simulink model "Final_motores"  (R2020b)
settings: Solver=VariableStepAuto  StartTime=0.0  StopTime=10.0  MinStep=2e-6  RelTol=1e-3
model workspace (MAT data in the model file):
  potencia = 0.1
values from neighbouring files (symbols this model uses):
  b = 1.5e-5    (= 1.5e-05)    [Var_PF.m]
  Jl = Jl/100^2/1000    (= 0.00048022)    [Var_PF.m]
  Ke = Ke*60/(2*pi)    (= 131.78029288)    [Var_PF.m]
  Kt = Kt/100    (= 0.133)    [Var_PF.m]
  La = 1.4/1000    (= 0.0014)    [Var_PF.m]
  Ra = 0.4    [Var_PF.m]
undefined symbols (not defined in the file or in its folder): B, ba, C_f, DiscIntNeverNeededParam, f_mues, gama, Ksa, Ksia, Kto, Kwo, mult, ohmega_obser, ohmega_pos, r, R, R_f, time_MV, Vmax_controlador, Vmax_salida, w_ia
libraries: dspfdesign x3, commchan3 x3, mcbcontrolslib x2, simulink x1, dspstat3 x1
settings Model: Creator=GoniR  LastModifiedBy=GoniR

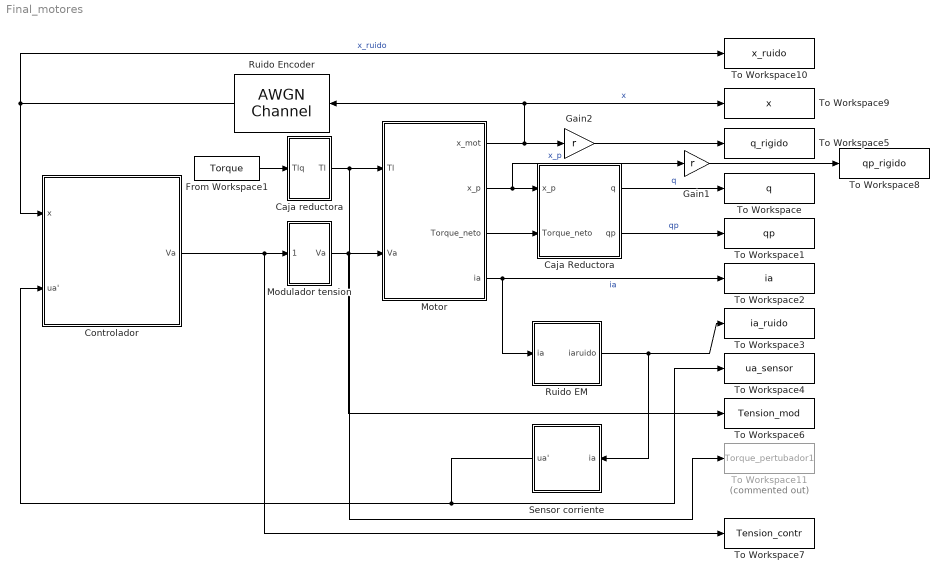
== system Final_motores ==
  Caja Reductora : Subsystem
  Caja reductora : Subsystem
  Controlador : Subsystem
  From Workspace1 : FromWorkspace  VariableName=Torque
  Gain1 : Gain  Gain=r
  Gain2 : Gain  Gain=r
  Modulador tension : Subsystem
  Motor : Subsystem
  Ruido EM : Subsystem
  Ruido Encoder : commchan3/AWGN Channel  InputProcessing=Columns as channels (frame based)  seed=67  noiseMode=Variance from mask  EbNodB=10  EsNodB=30  SNRdB=30  bitsPerSym=1  Ps=1  Tsym=1  variance=((1/(5000)*2*pi /360)/2)^2
  Sensor corriente : Subsystem
  To Workspace : ToWorkspace  VariableName=q  SaveFormat=Timeseries  SampleTime=-1
  To Workspace1 : ToWorkspace  VariableName=qp  SaveFormat=Timeseries  SampleTime=-1
  To Workspace10 : ToWorkspace  VariableName=x_ruido  SaveFormat=Timeseries  SampleTime=-1
  To Workspace11 : ToWorkspace  Commented=on  VariableName=Torque_pertubador1  SaveFormat=Timeseries  SampleTime=-1
  To Workspace2 : ToWorkspace  VariableName=ia  SaveFormat=Timeseries  SampleTime=-1
  To Workspace3 : ToWorkspace  VariableName=ia_ruido  SaveFormat=Timeseries  SampleTime=-1
  To Workspace4 : ToWorkspace  VariableName=ua_sensor  SaveFormat=Timeseries  SampleTime=-1
  To Workspace5 : ToWorkspace  VariableName=q_rigido  SaveFormat=Timeseries  SampleTime=-1
  To Workspace6 : ToWorkspace  VariableName=Tension_mod  SaveFormat=Timeseries  SampleTime=-1
  To Workspace7 : ToWorkspace  VariableName=Tension_contr  SaveFormat=Timeseries  SampleTime=-1
  To Workspace8 : ToWorkspace  VariableName=qp_rigido  SaveFormat=Timeseries  SampleTime=-1
  To Workspace9 : ToWorkspace  VariableName=x  SaveFormat=Timeseries  SampleTime=-1
  wires:
  Motor/4(ia) -> Ruido EM/1(ia), To Workspace2/1  "ia"
  Controlador/1(Va) -> To Workspace7/1, Modulador tension/1(Va*)
  Caja reductora/1(Tl) -> To Workspace11/1, Motor/1(Tl)
  Modulador tension/1(Va) -> To Workspace6/1, Motor/2(Va)
  Motor/2(x_p) -> Gain1/1, Caja Reductora/1(x_p)  "x_p"
  Sensor corriente/1(ua') -> Controlador/2(ua'), To Workspace4/1
  Caja Reductora/1(q) -> To Workspace/1  "q"
  Caja Reductora/2(qp) -> To Workspace1/1  "qp"
  Ruido EM/1(iaruido) -> Sensor corriente/1(ia), To Workspace3/1
  Motor/3(Torque_neto) -> Caja Reductora/2(Torque_neto)
  Motor/1(x_mot) -> Ruido Encoder/1, To Workspace9/1, Gain2/1  "x"
  Gain2/1 -> To Workspace5/1
  From Workspace1/1 -> Caja reductora/1(Tlq)
  Ruido Encoder/1 -> To Workspace10/1, Controlador/1(x)  "x_ruido"
  Gain1/1 -> To Workspace8/1

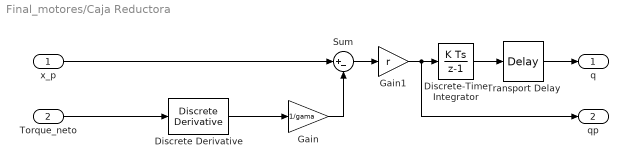
== system Final_motores/Caja Reductora ==
  x_p : Inport
  Torque_neto : Inport  Port=2
  Discrete Derivative : simulink/Discrete/Discrete Derivative  gainval=1.0  ICPrevScaledInput=0.0  OutMin=[]  OutMax=[]  OutDataType=fixdt(1, 16)  OutScaling=2^-10  DoSatur=off
  Discrete-Time Integrator : DiscreteIntegrator  SampleTime=-1  ICPrevOutput=DiscIntNeverNeededParam  ICPrevScaledInput=DiscIntNeverNeededParam
  Gain : Gain  Gain=1/gama
  Gain1 : Gain  Gain=r
  Sum : Sum  Inputs=|+-
  Transport Delay : TransportDelay  DelayTime=1e-6
  q : Outport
  qp : Outport  Port=2
  wires:
  Gain/1 -> Sum/2
  Torque_neto/1 -> Discrete Derivative/1
  Discrete Derivative/1 -> Gain/1
  x_p/1 -> Sum/1
  Sum/1 -> Gain1/1
  Discrete-Time Integrator/1 -> Transport Delay/1
  Transport Delay/1 -> q/1
  Gain1/1 -> qp/1, Discrete-Time Integrator/1

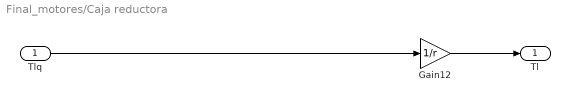
== system Final_motores/Caja reductora ==
  Tlq : Inport
  Gain12 : Gain  Gain=1/r
  Tl : Outport
  wires:
  Tlq/1 -> Gain12/1
  Gain12/1 -> Tl/1

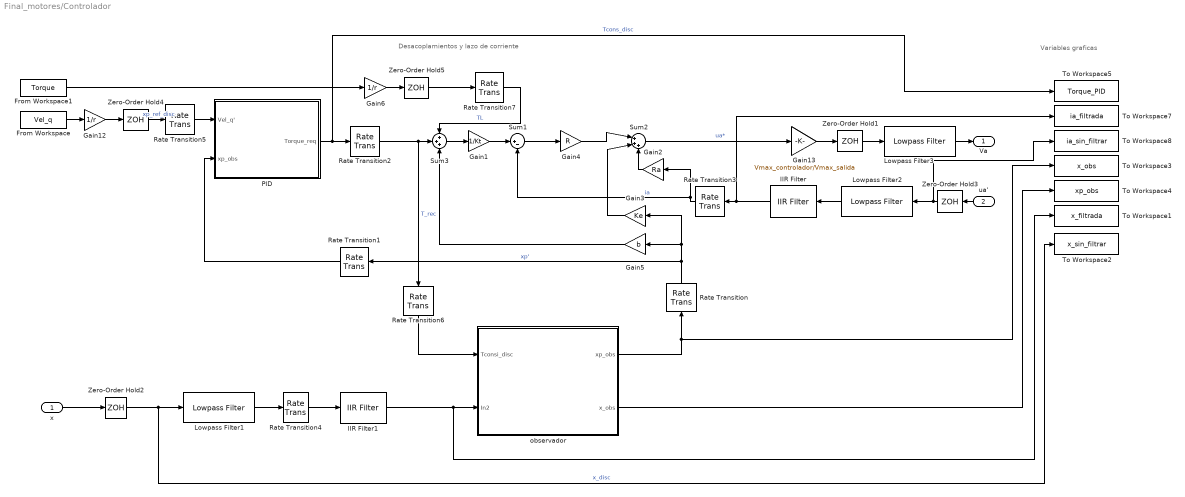
== system Final_motores/Controlador ==
  note: Desacoplamientos y lazo de corriente
  note: Variables graficas
  x : Inport
  ua' : Inport  Port=2
  From Workspace : FromWorkspace  VariableName=Vel_q
  From Workspace1 : FromWorkspace  VariableName=Torque
  Gain1 : Gain  Gain=1/Kt
  Gain12 : Gain  Gain=1/r
  Gain13 : Gain  Gain=Vmax_controlador/Vmax_salida
  Gain2 : Gain  Gain=Ra
  Gain3 : Gain  Gain=Ke
  Gain4 : Gain  Gain=R
  Gain5 : Gain  Gain=b
  Gain6 : Gain  Gain=1/r
  IIR Filter : mcbcontrolslib/IIR Filter  Filter_constant=0.01
      settings: SourceProductBaseCode=MT
  IIR Filter1 : mcbcontrolslib/IIR Filter  Filter_constant=0.01
      settings: SourceProductBaseCode=MT
  Lowpass Filter1 : dspfdesign/Lowpass Filter  FilterType=IIR  DesignForMinimumOrder=on  FilterOrder=50  PassbandFrequency=ohmega_obser*2  StopbandFrequency=ohmega_obser*2+1000  PassbandRipple=0.1  StopbandAttenuation=80  InheritSampleRate=on  SampleRate=44100  SimulateUsing=Interpreted execution  roundingMode=Floor  coeffsDataTypeStr=fixdt(1,16)
  Lowpass Filter2 : dspfdesign/Lowpass Filter  FilterType=IIR  DesignForMinimumOrder=on  FilterOrder=50  PassbandFrequency=2*w_ia  StopbandFrequency=2*w_ia+1000  PassbandRipple=0.1  StopbandAttenuation=80  InheritSampleRate=on  SampleRate=44100  SimulateUsing=Interpreted execution  roundingMode=Floor  coeffsDataTypeStr=fixdt(1,16)
  Lowpass Filter3 : dspfdesign/Lowpass Filter  FilterType=IIR  DesignForMinimumOrder=on  FilterOrder=50  PassbandFrequency=ohmega_obser*2  StopbandFrequency=ohmega_obser*2+1000  PassbandRipple=0.1  StopbandAttenuation=80  InheritSampleRate=on  SampleRate=44100  SimulateUsing=Interpreted execution  roundingMode=Floor  coeffsDataTypeStr=fixdt(1,16)
  PID : Subsystem
  Rate Transition{,2..3,7} (4 alike) : RateTransition  OutPortSampleTime=1/(w_ia*mult)
  Rate Transition1 : RateTransition  OutPortSampleTime=1/(ohmega_pos*mult)
  Rate Transition4 : RateTransition  OutPortSampleTime=1/(ohmega_obser*mult)
  Rate Transition5 : RateTransition  OutPortSampleTime=1/(ohmega_pos*mult)
  Rate Transition6 : RateTransition  OutPortSampleTime=1/(ohmega_obser*mult)
  Sum1 : Sum  Inputs=|+-
  Sum2 : Sum  Inputs=|+++
  Sum3 : Sum  Inputs=+++
  To Workspace1 : ToWorkspace  VariableName=x_filtrada  SaveFormat=Timeseries  SampleTime=-1
  To Workspace2 : ToWorkspace  VariableName=x_sin_filtrar  SaveFormat=Timeseries  SampleTime=-1
  To Workspace3 : ToWorkspace  VariableName=x_obs  SaveFormat=Timeseries  SampleTime=-1
  To Workspace4 : ToWorkspace  VariableName=xp_obs  SaveFormat=Timeseries  SampleTime=-1
  To Workspace5 : ToWorkspace  VariableName=Torque_PID  SaveFormat=Timeseries  SampleTime=-1
  To Workspace7 : ToWorkspace  VariableName=ia_filtrada  SaveFormat=Timeseries  SampleTime=-1
  To Workspace8 : ToWorkspace  VariableName=ia_sin_filtrar  SaveFormat=Timeseries  SampleTime=-1
  Zero-Order Hold{1..5} (5 alike) : ZeroOrderHold  SampleTime=1/f_mues
  observador : Subsystem
  Va : Outport
  wires:
  Sum3/1 -> Gain1/1
  Sum1/1 -> Gain4/1
  Gain2/1 -> Sum2/3
  Gain4/1 -> Sum2/1
  Gain3/1 -> Sum2/2
  Gain1/1 -> Sum1/1
  Sum2/1 -> Gain13/1  "ua*"
  Gain12/1 -> Zero-Order Hold4/1
  Gain13/1 -> Zero-Order Hold1/1
  ua'/1 -> Zero-Order Hold3/1
  PID/1(Torque_req) -> To Workspace5/1, Rate Transition2/1  "Tcons_disc"
  Zero-Order Hold4/1 -> Rate Transition5/1  "xp_ref_disc"
  observador/1(xp_obs) -> Rate Transition/1, To Workspace3/1
  Rate Transition/1 -> Rate Transition1/1, Gain3/1, Gain5/1  "xp'"
  Rate Transition1/1 -> PID/2(xp_obs)
  Rate Transition5/1 -> PID/1(Vel_q')
  Rate Transition6/1 -> observador/1(Tconsi_disc)
  Rate Transition3/1 -> Sum1/2, Gain2/1  "ia"
  From Workspace1/1 -> Gain6/1
  From Workspace/1 -> Gain12/1
  Zero-Order Hold5/1 -> Rate Transition7/1
  Gain6/1 -> Zero-Order Hold5/1
  x/1 -> Zero-Order Hold2/1
  IIR Filter1/1 -> To Workspace1/1, observador/2(In2)
  Rate Transition4/1 -> IIR Filter1/1
  Zero-Order Hold2/1 -> To Workspace2/1, Lowpass Filter1/1  "x_disc"
  Lowpass Filter1/1 -> Rate Transition4/1
  IIR Filter/1 -> To Workspace7/1, Rate Transition3/1
  observador/2(x_obs) -> To Workspace4/1
  Zero-Order Hold1/1 -> Lowpass Filter3/1
  Rate Transition2/1 -> Rate Transition6/1, Sum3/2  "T_rec"
  Gain5/1 -> Sum3/3
  Rate Transition7/1 -> Sum3/1  "TL"
  Zero-Order Hold3/1 -> To Workspace8/1, Lowpass Filter2/1
  Lowpass Filter2/1 -> IIR Filter/1
  Lowpass Filter3/1 -> Va/1

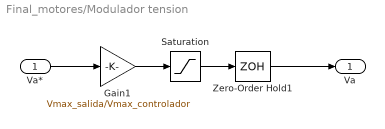
== system Final_motores/Modulador tension ==
  Va* : Inport
  Gain1 : Gain  Gain=Vmax_salida/Vmax_controlador
  Saturation : Saturate  UpperLimit=60  LowerLimit=-60
  Zero-Order Hold1 : ZeroOrderHold  SampleTime=time_MV
  Va : Outport
  wires:
  Va*/1 -> Gain1/1
  Gain1/1 -> Saturation/1
  Saturation/1 -> Zero-Order Hold1/1
  Zero-Order Hold1/1 -> Va/1

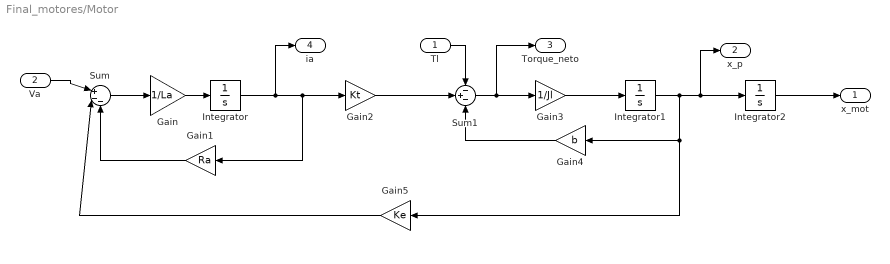
== system Final_motores/Motor ==
  Tl : Inport
  Va : Inport  Port=2
  Gain : Gain  Gain=1/La
  Gain1 : Gain  Gain=Ra
  Gain2 : Gain  Gain=Kt
  Gain3 : Gain  Gain=1/Jl
  Gain4 : Gain  Gain=b
  Gain5 : Gain  Gain=Ke
  Integrator : Integrator
  Integrator1 : Integrator
  Integrator2 : Integrator
  Sum : Sum  Inputs=|+--
  Sum1 : Sum  Inputs=-+-
  x_mot : Outport
  x_p : Outport  Port=2
  Torque_neto : Outport  Port=3
  ia : Outport  Port=4
  wires:
  Sum1/1 -> Torque_neto/1, Gain3/1
  Va/1 -> Sum/1
  Integrator2/1 -> x_mot/1
  Integrator/1 -> ia/1, Gain2/1, Gain1/1
  Gain/1 -> Integrator/1
  Gain3/1 -> Integrator1/1
  Gain2/1 -> Sum1/2
  Sum/1 -> Gain/1
  Integrator1/1 -> x_p/1, Integrator2/1, Gain5/1, Gain4/1
  Gain4/1 -> Sum1/3
  Gain1/1 -> Sum/3
  Gain5/1 -> Sum/2
  Tl/1 -> Sum1/1

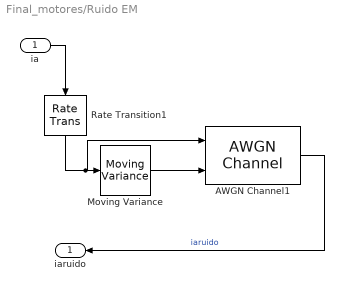
== system Final_motores/Ruido EM ==
  ia : Inport
  AWGN Channel1 : commchan3/AWGN Channel  InputProcessing=Columns as channels (frame based)  seed=67  noiseMode=Variance from port  EbNodB=10  EsNodB=30  SNRdB=30  bitsPerSym=1  Ps=1  Tsym=1  variance=5^2/0.045^2
  Moving Variance : dspstat3/Moving Variance  Method=Sliding window  ForgettingFactorPort=off  SpecifyWindowLength=on  WindowLength=50  ForgettingFactor=0.9  SimulateUsing=Code generation
      settings: SourceProductBaseCode=DS
  Rate Transition1 : RateTransition  OutPortSampleTime=1/(w_ia*25)
  iaruido : Outport
  wires:
  Rate Transition1/1 -> AWGN Channel1/1, Moving Variance/1
  ia/1 -> Rate Transition1/1
  AWGN Channel1/1 -> iaruido/1  "iaruido"
  Moving Variance/1 -> AWGN Channel1/2

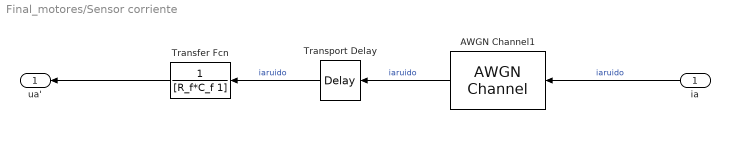
== system Final_motores/Sensor corriente ==
  ia : Inport
  AWGN Channel1 : commchan3/AWGN Channel  InputProcessing=Columns as channels (frame based)  seed=5  noiseMode="Signal to noise ratio  (SNR)"  EbNodB=10  EsNodB=5^2/0.045^2  SNRdB=log10(2100^2)-log10(0.045^2)  bitsPerSym=1  Ps=0.1  Tsym=1  variance=5^2/0.045^2
  Transfer Fcn : TransferFcn  Denominator=[R_f*C_f 1]
  Transport Delay : TransportDelay  DelayTime=1e-6
  ua' : Outport
  wires:
  ia/1 -> AWGN Channel1/1  "iaruido"
  AWGN Channel1/1 -> Transport Delay/1  "iaruido"
  Transfer Fcn/1 -> ua'/1
  Transport Delay/1 -> Transfer Fcn/1  "iaruido"

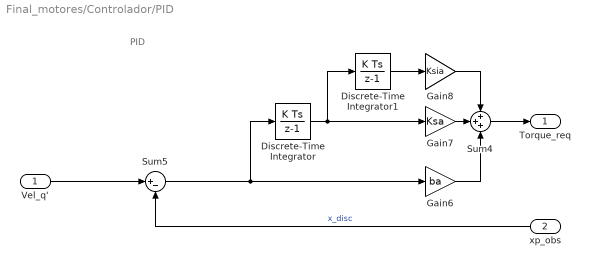
== system Final_motores/Controlador/PID ==
  note: PID
  Vel_q' : Inport
  xp_obs : Inport  Port=2
  Discrete-Time Integrator : DiscreteIntegrator  SampleTime=-1  ICPrevOutput=DiscIntNeverNeededParam  ICPrevScaledInput=DiscIntNeverNeededParam
  Discrete-Time Integrator1 : DiscreteIntegrator  SampleTime=-1  ICPrevOutput=DiscIntNeverNeededParam  ICPrevScaledInput=DiscIntNeverNeededParam
  Gain6 : Gain  Gain=ba
  Gain7 : Gain  Gain=Ksa
  Gain8 : Gain  Gain=Ksia
  Sum4 : Sum  Inputs=+++
  Sum5 : Sum  Inputs=|+-
  Torque_req : Outport
  wires:
  Sum4/1 -> Torque_req/1
  Gain8/1 -> Sum4/1
  Gain6/1 -> Sum4/3
  Discrete-Time Integrator/1 -> Discrete-Time Integrator1/1, Gain7/1
  Gain7/1 -> Sum4/2
  Discrete-Time Integrator1/1 -> Gain8/1
  Vel_q'/1 -> Sum5/1
  xp_obs/1 -> Sum5/2  "x_disc"
  Sum5/1 -> Gain6/1, Discrete-Time Integrator/1

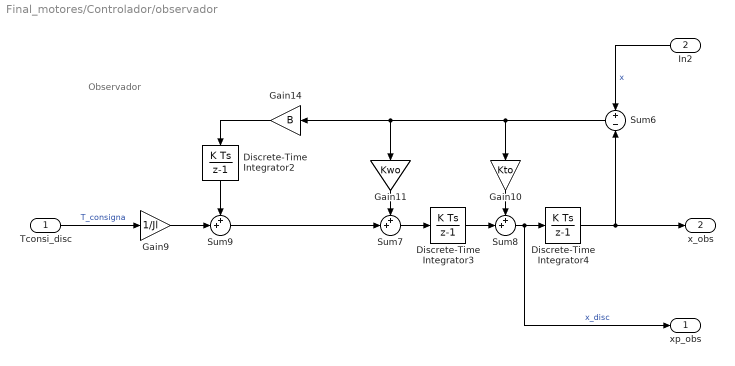
== system Final_motores/Controlador/observador ==
  note: Observador
  Tconsi_disc : Inport
  In2 : Inport  Port=2
  Discrete-Time Integrator2 : DiscreteIntegrator  SampleTime=-1  ICPrevOutput=DiscIntNeverNeededParam  ICPrevScaledInput=DiscIntNeverNeededParam
  Discrete-Time Integrator3 : DiscreteIntegrator  SampleTime=-1  ICPrevOutput=DiscIntNeverNeededParam  ICPrevScaledInput=DiscIntNeverNeededParam
  Discrete-Time Integrator4 : DiscreteIntegrator  SampleTime=-1  ICPrevOutput=DiscIntNeverNeededParam  ICPrevScaledInput=DiscIntNeverNeededParam
  Gain10 : Gain  Gain=Kto
  Gain11 : Gain  Gain=Kwo
  Gain14 : Gain  Gain=B
  Gain9 : Gain  Gain=1/Jl
  Sum6 : Sum  Inputs=+|-
  Sum7 : Sum  Inputs=++|
  Sum8 : Sum  Inputs=++|
  Sum9 : Sum  Inputs=++|
  xp_obs : Outport
  x_obs : Outport  Port=2
  wires:
  Gain10/1 -> Sum8/1
  Sum9/1 -> Sum7/2
  Discrete-Time Integrator4/1 -> Sum6/2, x_obs/1
  Gain11/1 -> Sum7/1
  Gain14/1 -> Discrete-Time Integrator2/1
  Discrete-Time Integrator3/1 -> Sum8/2
  Sum6/1 -> Gain10/1, Gain11/1, Gain14/1
  Discrete-Time Integrator2/1 -> Sum9/1
  Sum7/1 -> Discrete-Time Integrator3/1
  Tconsi_disc/1 -> Gain9/1  "T_consigna"
  In2/1 -> Sum6/1  "x"
  Sum8/1 -> xp_obs/1, Discrete-Time Integrator4/1  "x_disc"
  Gain9/1 -> Sum9/2
